simulink model "Lab1_Encoder_24"  (R2024b)
settings: Solver=FixedStepAuto  StartTime=0.0  StopTime=inf  FixedStep=0.01  RelTol=1e-3  EnableMultiTasking=on
libraries: stm32f4xxblockslib x4, stm32g4xxblockslib x3
settings Model: STM32="{\"DigitalPortRead\":[{\"ID\":\"Lab1_Encoder_24:6\"},{\"ID\":\"Lab1_Encoder_24:7\"},{\"ID\":\"Lab1_Encoder_24:8\"},{\"ID\":\"Lab1_Encoder_24:9\"}],\"EncoderBlockForG4\":[{\"ID\":\"Lab1_Encoder_24:30\"},{\"ID\":\"Lab1_Encoder_24:31\"},{\"ID\":\"Lab1_Encoder_24:32\"}]}"  Creator=Aom  LastModifiedBy=Aom
settings OptimizationCC: DefaultParameterBehavior=Inlined  EnhancedBackFolding=on  PassReuseOutputArgsAs=Individual arguments  ZeroExternalMemoryAtStartup=off  ZeroInternalMemoryAtStartup=off  MaxStackSize=512  OptimizeBlockOrder=speed  DifferentSizesBufferReuse=on  OptimizationCustomize=off  EfficientTunableParamExpr=on
settings DebuggingCC: ParameterTunabilityLossMsg=error
settings HardwareCC: ProdBitPerPointer=32  ProdBitPerSizeT=32  ProdBitPerPtrDiffT=32  ProdLargestAtomicInteger=Long  ProdLargestAtomicFloat=Double  ProdWordSize=32  ProdLongLongMode=on  ProdHWDeviceType=ARM Compatible->ARM Cortex-M
settings SFSimCC: MATLABDynamicMemAlloc=off
settings RTWCC: Description=Embedded Coder  SystemTargetFile=ert.tlc  HardwareBoard=STM32G4xx Based  TemplateMakefile=ert_default_tmf  Toolchain=GNU Tools for ARM Embedded Processors
settings CodeAppCC: ForceParamTrailComments=on  IgnoreCustomStorageClasses=off  OperatorAnnotations=on  SimulinkDataObjDesc=on  SFDataObjDesc=on  InsertBlockDesc=on
settings ERTTargetCC: TargetLangStandard=C99 (ISO)  CodeReplacementLibrary=ARM Cortex-M  ExtModeTransport=3  ExtModeStaticAlloc=on  ExtModeStaticAllocSize=2048  ExtModeMexFile=ext_xcp  ExtModeIntrfLevel=Level2 - Open

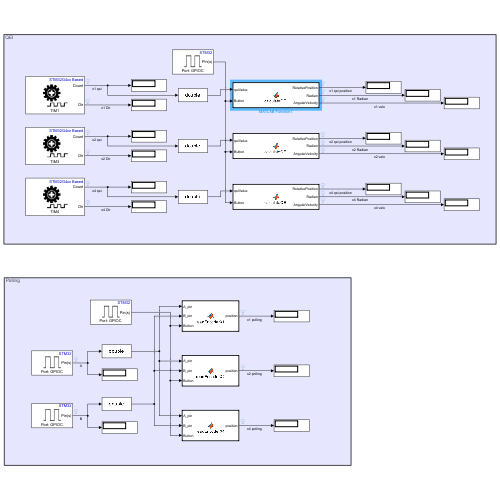
[thumbnail: Simulink's stored preview of the top-level diagram]
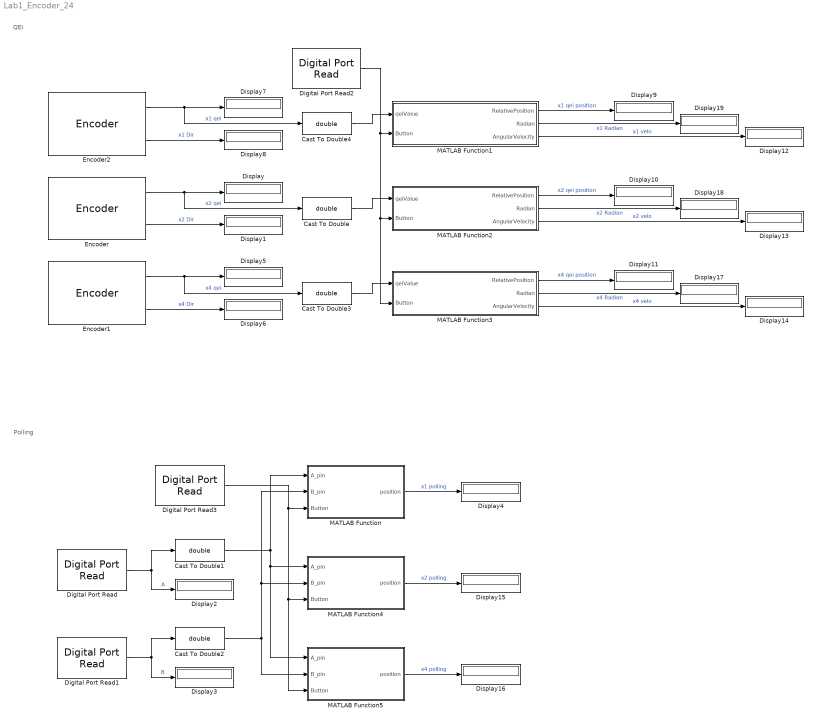
== system Lab1_Encoder_24 ==
  note: Polling
  note: QEI
  Cast To Double{,1..4} (5 alike) : DataTypeConversion  OutDataTypeStr=double  SaturateOnIntegerOverflow=off  RndMeth=Floor
  Digital Port Read : stm32f4xxblockslib/Digital Port Read  PortName=GPIOC  PinNumber=2  ReadOperation=on  IOAsArray=on  SampleTime=-1  EnableSimPort=off  hoistedMaskSrc=ECSoC/ECSimCodegen/Digital Port Read
      settings: LibrarySourceBlock=stm32g4xxblockslib/Digital Port Read
  Digital Port Read1 : stm32f4xxblockslib/Digital Port Read  PortName=GPIOC  PinNumber=3  ReadOperation=on  IOAsArray=on  SampleTime=-1  EnableSimPort=off  hoistedMaskSrc=ECSoC/ECSimCodegen/Digital Port Read
      settings: LibrarySourceBlock=stm32g4xxblockslib/Digital Port Read
  Digital Port Read2 : stm32f4xxblockslib/Digital Port Read  PortName=GPIOC  PinNumber=13  ReadOperation=on  IOAsArray=on  SampleTime=-1  EnableSimPort=off  hoistedMaskSrc=ECSoC/ECSimCodegen/Digital Port Read
      settings: LibrarySourceBlock=stm32g4xxblockslib/Digital Port Read
  Digital Port Read3 : stm32f4xxblockslib/Digital Port Read  PortName=GPIOC  PinNumber=13  ReadOperation=on  IOAsArray=on  SampleTime=-1  EnableSimPort=off  hoistedMaskSrc=ECSoC/ECSimCodegen/Digital Port Read
      settings: LibrarySourceBlock=stm32g4xxblockslib/Digital Port Read
  Display{,1..19} (20 alike) : Display
  Encoder : stm32g4xxblockslib/Encoder  TimerModule=TIM3  EnableResetInput=off  OutputCountAfterFirstIndex=off  OutputValidIndex=off  OutputDirection=on  OutputStatus=off  SampleTime=-1
  Encoder1 : stm32g4xxblockslib/Encoder  TimerModule=TIM4  EnableResetInput=off  OutputCountAfterFirstIndex=off  OutputValidIndex=off  OutputDirection=on  OutputStatus=off  SampleTime=-1
  Encoder2 : stm32g4xxblockslib/Encoder  TimerModule=TIM1  EnableResetInput=off  OutputCountAfterFirstIndex=off  OutputValidIndex=off  OutputDirection=on  OutputStatus=off  SampleTime=-1
  MATLAB Function : MATLAB Function  TreatAsAtomicUnit=on
  MATLAB Function1 : MATLAB Function  TreatAsAtomicUnit=on
  MATLAB Function2 : MATLAB Function  TreatAsAtomicUnit=on
  MATLAB Function3 : MATLAB Function  TreatAsAtomicUnit=on
  MATLAB Function4 : MATLAB Function  TreatAsAtomicUnit=on
  MATLAB Function5 : MATLAB Function  TreatAsAtomicUnit=on
  wires:
  MATLAB Function2/2(Radian) -> Display18/1  "x2 Radian"
  MATLAB Function1/3(AngularVelocity) -> Display12/1  "x1 velo"
  MATLAB Function4/1(position) -> Display15/1  "x2 polling"
  MATLAB Function1/2(Radian) -> Display19/1  "x1 Radian"
  Digital Port Read2/1 -> MATLAB Function2/2(Button), MATLAB Function3/2(Button), MATLAB Function1/2(Button)
  Encoder1/1 -> Cast To Double3/1, Display5/1  "x4 qei"
  Encoder1/2 -> Display6/1  "x4 Dir"
  Digital Port Read3/1 -> MATLAB Function/3(Button), MATLAB Function4/3(Button), MATLAB Function5/3(Button)
  MATLAB Function2/3(AngularVelocity) -> Display13/1  "x2 velo"
  Encoder2/2 -> Display8/1  "x1 Dir"
  Encoder/1 -> Cast To Double/1, Display/1  "x2 qei"
  Encoder2/1 -> Cast To Double4/1, Display7/1  "x1 qei"
  MATLAB Function5/1(position) -> Display16/1  "x4 polling"
  Digital Port Read1/1 -> Cast To Double2/1, Display3/1  "B"
  MATLAB Function2/1(RelativePosition) -> Display10/1  "x2 qei position"
  Cast To Double4/1 -> MATLAB Function1/1(qeiValue)
  Cast To Double/1 -> MATLAB Function2/1(qeiValue)
  Cast To Double3/1 -> MATLAB Function3/1(qeiValue)
  Digital Port Read/1 -> Cast To Double1/1, Display2/1  "A"
  MATLAB Function3/3(AngularVelocity) -> Display14/1  "x4 velo"
  Cast To Double1/1 -> MATLAB Function/1(A_pin), MATLAB Function4/1(A_pin), MATLAB Function5/1(A_pin)
  Encoder/2 -> Display1/1  "x2 Dir"
  Cast To Double2/1 -> MATLAB Function/2(B_pin), MATLAB Function4/2(B_pin), MATLAB Function5/2(B_pin)
  MATLAB Function3/1(RelativePosition) -> Display11/1  "x4 qei position"
  MATLAB Function1/1(RelativePosition) -> Display9/1  "x1 qei position"
  MATLAB Function/1(position) -> Display4/1  "x1 polling"
  MATLAB Function3/2(Radian) -> Display17/1  "x4 Radian"

== matlab function Lab1_Encoder_24/MATLAB Function1 ==
  data: qeiValue input; RelativePosition output; Radian output; Button input; AngularVelocity output
function [RelativePosition, Radian, AngularVelocity] = calculateQEI(qeiValue, Button)
    % Maximum QEI counter
    maxQEIValue = 65520;
    
    % Resolution of the encoder
    encoderResolution = 24;

    % x1
    encoderResolution = encoderResolution * 1;
    
    % Fixed-step time of 0.01 seconds
    fixedStepSize = 0.01; 
    
    % Persistent variables
    persistent prevQEIValue signedCount prevSignedCount;
    
    % Initialize persistent variables if they are empty
    if isempty(prevQEIValue)
        prevQEIValue = qeiValue;
        signedCount = 0;
        prevSignedCount = 0;
    end
    
    % Difference between current and previous QEI values
    delta = qeiValue - prevQEIValue;
    
    % Reset
    if Button == 1
        signedCount = 0;
    end

    % Detect wrap-around conditions and adjust the signed count accordingly
    if delta > maxQEIValue / 2
        % Counter wrapped from 0 to maxQEIValue
        signedCount = signedCount - (maxQEIValue - delta + 1);
    elseif delta < -maxQEIValue / 2
        % Counter wrapped from maxQEIValue to 0
        signedCount = signedCount + (maxQEIValue + delta + 1);
    else
        % Normal counting
        signedCount = signedCount + delta;
    end
    
    % Calculate the change in signed position (AngularVelocity in counts per step)
    AngularVelo = signedCount - prevSignedCount;
    
    % Calculate AngularVelocity in terms of radians per second
    AngularVelo = AngularVelo / fixedStepSize;
    AngularVelo = (AngularVelo / encoderResolution) * 2 * pi;

    % Update the previous QEI value and signed count
    prevQEIValue = qeiValue;
    prevSignedCount = signedCount;
    
    % Output the signed position in counts
    RelativePosition = signedCount;

    % Output the Radian
    Radian = (signedCount / encoderResolution) * 2 * pi;
    
    % Output the integrated distance in revolutions
    AngularVelocity = AngularVelo;
end

== matlab function Lab1_Encoder_24/MATLAB Function ==
  data: A_pin input; B_pin input; position output; Button input
function position = readEncoderX1(A_pin, B_pin, Button)
    % Define persistent variables
    persistent prevState pos;
    
    % Initialize persistent variables if they are empty
    if isempty(prevState)
        prevState = 0;
        pos = 0;
    end

    % Read the current state of the encoder pins A and B
    currentStateA = A_pin;
    currentStateB = B_pin;

    % Reset position if the button is pressed
    if Button == 1
        pos = 0;
    end

    % Detect rising edge of A_pin to count
    if (prevState == 0) && (currentStateA == 1)
        % Check direction based on the state of B pin
        if currentStateB == 0
            pos = pos + 1;
        else
            pos = pos - 1;
        end
    end

    % Update the previous state of A_pin
    prevState = currentStateA;

    % Output the position
    position = pos;
end

== matlab function Lab1_Encoder_24/MATLAB Function2 ==
  data: qeiValue input; RelativePosition output; Radian output; Button input; AngularVelocity output
function [RelativePosition, Radian, AngularVelocity] = calculateQEI(qeiValue, Button)
    % Maximum QEI counter
    maxQEIValue = 65520;
    
    % Resolution of the encoder
    encoderResolution = 24;

    % x2
    encoderResolution = encoderResolution * 2;
    
    % Fixed-step time of 0.01 seconds
    fixedStepSize = 0.01; 
    
    % Persistent variables
    persistent prevQEIValue signedCount prevSignedCount;
    
    % Initialize persistent variables if they are empty
    if isempty(prevQEIValue)
        prevQEIValue = qeiValue;
        signedCount = 0;
        prevSignedCount = 0;
    end
    
    % Difference between current and previous QEI values
    delta = qeiValue - prevQEIValue;
    
    % Reset
    if Button == 1
        signedCount = 0;
    end

    % Detect wrap-around conditions and adjust the signed count accordingly
    if delta > maxQEIValue / 2
        % Counter wrapped from 0 to maxQEIValue
        signedCount = signedCount - (maxQEIValue - delta + 1);
    elseif delta < -maxQEIValue / 2
        % Counter wrapped from maxQEIValue to 0
        signedCount = signedCount + (maxQEIValue + delta + 1);
    else
        % Normal counting
        signedCount = signedCount + delta;
    end
    
    % Calculate the change in signed position (AngularVelocity in counts per step)
    AngularVelo = signedCount - prevSignedCount;
    
    % Calculate AngularVelocity in terms of radians per second
    AngularVelo = AngularVelo / fixedStepSize;
    AngularVelo = (AngularVelo / encoderResolution) * 2 * pi;

    % Update the previous QEI value and signed count
    prevQEIValue = qeiValue;
    prevSignedCount = signedCount;
    
    % Output the signed position in counts
    RelativePosition = signedCount;
    
    % Output the Radian
    Radian = (signedCount / encoderResolution) * 2 * pi;

    % Output the integrated distance in revolutions
    AngularVelocity = AngularVelo;
end

== matlab function Lab1_Encoder_24/MATLAB Function3 ==
  data: qeiValue input; RelativePosition output; Radian output; Button input; AngularVelocity output
function [RelativePosition, Radian, AngularVelocity] = calculateQEI(qeiValue, Button)
    % Maximum QEI counter
    maxQEIValue = 65472;
    
    % Resolution of the encoder
    encoderResolution = 24;

    % x4
    encoderResolution = encoderResolution * 4;
    
    % Fixed-step time of 0.01 seconds
    fixedStepSize = 0.01; 
    
    % Persistent variables
    persistent prevQEIValue signedCount prevSignedCount;
    
    % Initialize persistent variables if they are empty
    if isempty(prevQEIValue)
        prevQEIValue = qeiValue;
        signedCount = 0;
        prevSignedCount = 0;
    end
    
    % Difference between current and previous QEI values
    delta = qeiValue - prevQEIValue;
    
    % Reset
    if Button == 1
        signedCount = 0;
    end

    % Detect wrap-around conditions and adjust the signed count accordingly
    if delta > maxQEIValue / 2
        % Counter wrapped from 0 to maxQEIValue
        signedCount = signedCount - (maxQEIValue - delta + 1);
    elseif delta < -maxQEIValue / 2
        % Counter wrapped from maxQEIValue to 0
        signedCount = signedCount + (maxQEIValue + delta + 1);
    else
        % Normal counting
        signedCount = signedCount + delta;
    end
    
    % Calculate the change in signed position (AngularVelocity in counts per step)
    AngularVelo = signedCount - prevSignedCount;
    
    % Calculate AngularVelocity in terms of radians per second
    AngularVelo = AngularVelo / fixedStepSize;
    AngularVelo = (AngularVelo / encoderResolution) * 2 * pi;

    % Update the previous QEI value and signed count
    prevQEIValue = qeiValue;
    prevSignedCount = signedCount;
    
    % Output the signed position in counts
    RelativePosition = signedCount;

    % Output the Radian
    Radian = (signedCount / encoderResolution) * 2 * pi;
    
    % Output the integrated distance in revolutions
    AngularVelocity = AngularVelo;
end

== matlab function Lab1_Encoder_24/MATLAB Function4 ==
  data: A_pin input; B_pin input; position output; Button input
function position = readEncoderX2(A_pin, B_pin, Button)
    % Define persistent variables
    persistent prevState pos;
    
    % Initialize persistent variables if they are empty
    if isempty(prevState)
        prevState = 0;
        pos = 0;
    end

    % Read the current state of the encoder pins A and B
    currentStateA = A_pin;
    currentStateB = B_pin;

    % Reset position if the button is pressed
    if Button == 1
        pos = 0;
    end

    % Detect both rising and falling edges of A_pin to count
    if (prevState == 0 && currentStateA == 1)  % Rising edge detection
        % Check direction based on the state of B pin
        if currentStateB == 0
            pos = pos + 1;
        else
            pos = pos - 1;
        end
    elseif (prevState == 1 && currentStateA == 0)  % Falling edge detection
        % Check direction based on the state of B pin
        if currentStateB == 1
            pos = pos + 1;
        else
            pos = pos - 1;
        end
    end

    % Update the previous state of A_pin
    prevState = currentStateA;

    % Output the position
    position = pos;
end

== matlab function Lab1_Encoder_24/MATLAB Function5 ==
  data: A_pin input; B_pin input; position output; Button input
function position = readEncoderX4(A_pin, B_pin, Button)
    % Define persistent variables
    persistent prevA prevB pos;
    
    % Initialize persistent variables if they are empty
    if isempty(prevA)
        prevA = 0;
        prevB = 0;
        pos = 0;
    end

    % Read the current state of the encoder pins A and B
    currentA = A_pin;
    currentB = B_pin;

    % Reset position if the button is pressed
    if Button == 1
        pos = 0;
    end

    % Determine direction and count based on all transitions (x4 mode)
    if (prevA == 0 && currentA == 1)  % Rising edge of A
        if currentB == 0
            pos = pos + 1;
        else
            pos = pos - 1;
        end
    elseif (prevA == 1 && currentA == 0)  % Falling edge of A
        if currentB == 1
            pos = pos + 1;
        else
            pos = pos - 1;
        end
    elseif (prevB == 0 && currentB == 1)  % Rising edge of B
        if currentA == 1
            pos = pos + 1;
        else
            pos = pos - 1;
        end
    elseif (prevB == 1 && currentB == 0)  % Falling edge of B
        if currentA == 0
            pos = pos + 1;
        else
            pos = pos - 1;
        end
    end

    % Update the previous states of A and B pins
    prevA = currentA;
    prevB = currentB;

    % Output the position
    position = pos;
end
